simulink model "PMSM_Drive_custom_pwm_discrete"  (R2019b)
settings: Solver=VariableStepAuto  StartTime=0.0  StopTime=0.5  MaxStep=1e-6  RelTol=1e-3
undefined symbols (not defined in the file): Apd, f_sw, Tid, U_DC
libraries: coordinate_transformations x4, simulink x2, PE_components x1, controllers x1
settings Model: SimulationMode=accelerator  Creator=kissd  LastModifiedBy=kissd

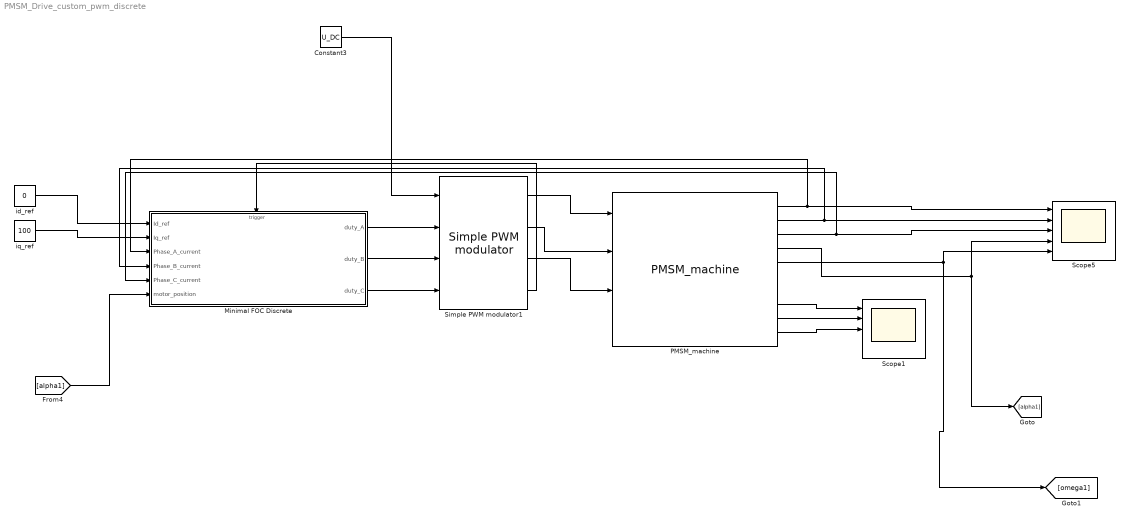
== system PMSM_Drive_custom_pwm_discrete ==
  Constant3 : Constant  Value=U_DC
  Minimal FOC Discrete : Subsystem  AncestorBlock=controllers/Minimal FOC Discrete
  PMSM_machine : PE_components/PMSM_machine  SystemSampleTime=-1  Latency=0  AutoFrameSizeCalculation=off
      link override Gain: Gain=1/Ld
      link override Gain1: Gain=Rs
      link override Gain2: Gain=Rs
      link override Gain4: Gain=1/Theta
      link override Gain7: Gain=3/2
      link override Integrator2: InitialCondition=0
      link override Sum2: Inputs=++-
  Scope1 : Scope  NumInputPorts=5
  Scope5 : Scope  NumInputPorts=5
  Simple PWM modulator1 : controllers/Simple PWM modulator  SystemSampleTime=-1  Latency=0  AutoFrameSizeCalculation=off
      link override Constant: Value=400
  id_ref : Constant  Value=0
  iq_ref : Constant  Value=100
  wires:
  PMSM_machine/2 -> Minimal FOC Discrete/4(Phase_B_current), Scope5/2
  PMSM_machine/3 -> Minimal FOC Discrete/5(Phase_C_current), Scope5/3
  PMSM_machine/1 -> Minimal FOC Discrete/3(Phase_A_current), Scope5/1
  PMSM_machine/4 -> [alpha1], Scope5/4
  PMSM_machine/5 -> [omega1], Scope5/5
  Constant3/1 -> Simple PWM modulator1/1
  Simple PWM modulator1/1 -> PMSM_machine/1
  Simple PWM modulator1/2 -> PMSM_machine/2
  Simple PWM modulator1/3 -> PMSM_machine/3
  PMSM_machine/8 -> Scope1/1
  PMSM_machine/9 -> Scope1/2
  PMSM_machine/10 -> Scope1/3
  id_ref/1 -> Minimal FOC Discrete/1(Id_ref)
  iq_ref/1 -> Minimal FOC Discrete/2(Iq_ref)
  [alpha1] -> Minimal FOC Discrete/6(motor_position)
  Minimal FOC Discrete/1(duty_A) -> Simple PWM modulator1/2
  Minimal FOC Discrete/2(duty_B) -> Simple PWM modulator1/3
  Minimal FOC Discrete/3(duty_C) -> Simple PWM modulator1/4
  Simple PWM modulator1/4 -> Minimal FOC Discrete/Trigger

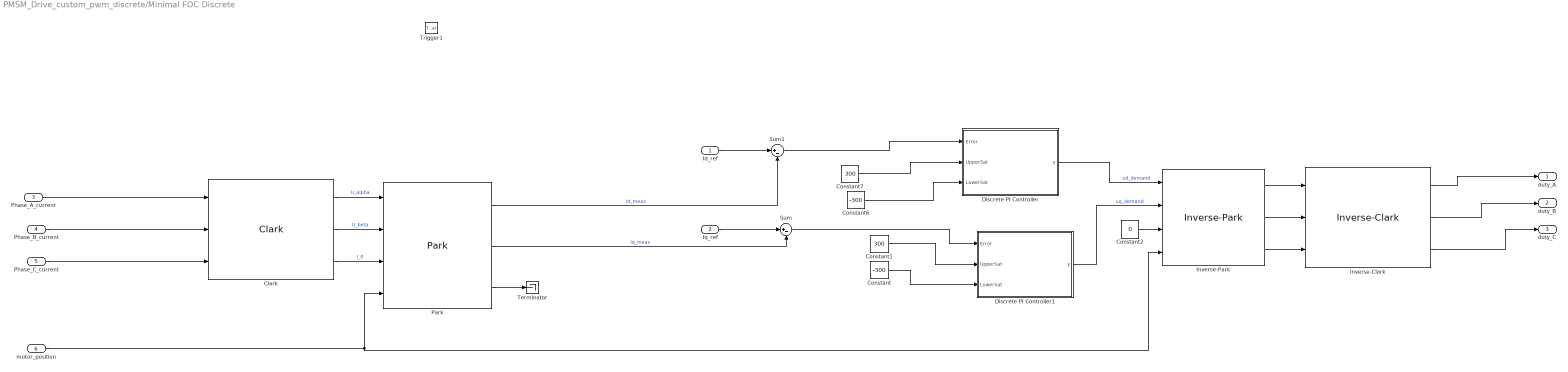
== system PMSM_Drive_custom_pwm_discrete/Minimal FOC Discrete ==
  Id_ref : Inport
  Iq_ref : Inport  Port=2
  Phase_A_current : Inport  Port=3
  Phase_B_current : Inport  Port=4
  Phase_C_current : Inport  Port=5
  motor_position : Inport  Port=6
  Trigger1 : TriggerPort  TriggerType=either  VariantControl=Variant  PortDimensions=1
  Clark : coordinate_transformations/Clark  SystemSampleTime=-1  Latency=0  AutoFrameSizeCalculation=off
  Constant : Constant  Value=-300
  Constant1 : Constant  Value=300
  Constant2 : Constant  Value=0
  Constant6 : Constant  Value=-300
  Constant7 : Constant  Value=300
  Discrete PI Controller : Subsystem  AncestorBlock=controllers/Discrete PI Controller  mask(Continous PI Controller){Apd=Apd, Tid=Tid, fs=f_sw}
      mask prompts: Apd "Proprotional Gain"; Tid "Integration Time"; fs "fsw"
      mask help: Continous PI Controller description.
  Discrete PI Controller1 : Subsystem  AncestorBlock=controllers/Discrete PI Controller  mask(Continous PI Controller){Apd=Apd, Tid=Tid, fs=f_sw}
      mask prompts: Apd "Proprotional Gain"; Tid "Integration Time"; fs "fsw"
      mask help: Continous PI Controller description.
  Inverse-Clark : coordinate_transformations/Inverse-Clark  SystemSampleTime=-1  Latency=0  AutoFrameSizeCalculation=off
  Inverse-Park : coordinate_transformations/Inverse-Park  SystemSampleTime=-1  Latency=0  AutoFrameSizeCalculation=off
  Park : coordinate_transformations/Park  SystemSampleTime=-1  Latency=0  AutoFrameSizeCalculation=off
  Sum : Sum  Inputs=|+-
  Sum1 : Sum  Inputs=|+-
  Terminator : Terminator
  duty_A : Outport
  duty_B : Outport  Port=2
  duty_C : Outport  Port=3
  wires:
  Discrete PI Controller1/1(y) -> Inverse-Park/2  "uq_demand"
  Inverse-Park/2 -> Inverse-Clark/2
  Inverse-Park/3 -> Inverse-Clark/3
  Park/2 -> Sum/2  "Iq_meas"
  Phase_C_current/1 -> Clark/3
  Constant7/1 -> Discrete PI Controller/2(UpperSat)
  Clark/1 -> Park/1  "U_alpha"
  Inverse-Clark/3 -> duty_C/1
  Constant1/1 -> Discrete PI Controller1/2(UpperSat)
  Sum/1 -> Discrete PI Controller1/1(Error)
  Inverse-Park/1 -> Inverse-Clark/1
  Constant6/1 -> Discrete PI Controller/3(LowerSat)
  motor_position/1 -> Park/4, Inverse-Park/4
  Park/1 -> Sum1/2  "Id_meas"
  Discrete PI Controller/1(y) -> Inverse-Park/1  "ud_demand"
  Constant/1 -> Discrete PI Controller1/3(LowerSat)
  Sum1/1 -> Discrete PI Controller/1(Error)
  Clark/2 -> Park/2  "U_beta"
  Iq_ref/1 -> Sum/1
  Clark/3 -> Park/3  "I_0"
  Park/3 -> Terminator/1
  Inverse-Clark/2 -> duty_B/1
  Id_ref/1 -> Sum1/1
  Inverse-Clark/1 -> duty_A/1
  Phase_B_current/1 -> Clark/2
  Phase_A_current/1 -> Clark/1
  Constant2/1 -> Inverse-Park/3

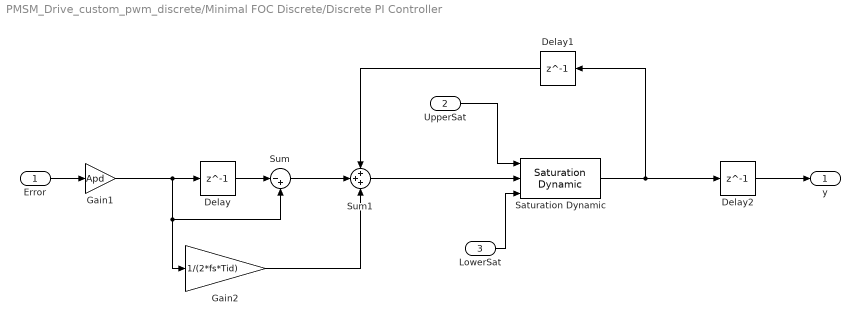
== system PMSM_Drive_custom_pwm_discrete/Minimal FOC Discrete/Discrete PI Controller ==
  Error : Inport
  UpperSat : Inport  Port=2
  LowerSat : Inport  Port=3
  Delay : Delay  DelayLength=1
  Delay1 : Delay  DelayLength=1
  Delay2 : Delay  DelayLength=1
  Gain1 : Gain  Gain=Apd
  Gain2 : Gain  Gain=1/(2*fs*Tid)
  Saturation Dynamic : simulink/Discontinuities/Saturation Dynamic  OutMin=[]  OutMax=[]  OutDataTypeStr=Inherit: Same as second input  OutDataType=fixdt(1, 16)  OutScaling=2^-10  DoSatur=off
  Sum : Sum  Inputs=|-+
  Sum1 : Sum  Inputs=+++
  y : Outport
  wires:
  Delay2/1 -> y/1
  Delay1/1 -> Sum1/1
  Gain2/1 -> Sum1/3
  Sum/1 -> Sum1/2
  Delay/1 -> Sum/1
  LowerSat/1 -> Saturation Dynamic/3
  UpperSat/1 -> Saturation Dynamic/1
  Saturation Dynamic/1 -> Delay2/1, Delay1/1
  Sum1/1 -> Saturation Dynamic/2
  Gain1/1 -> Delay/1, Sum/2, Gain2/1
  Error/1 -> Gain1/1

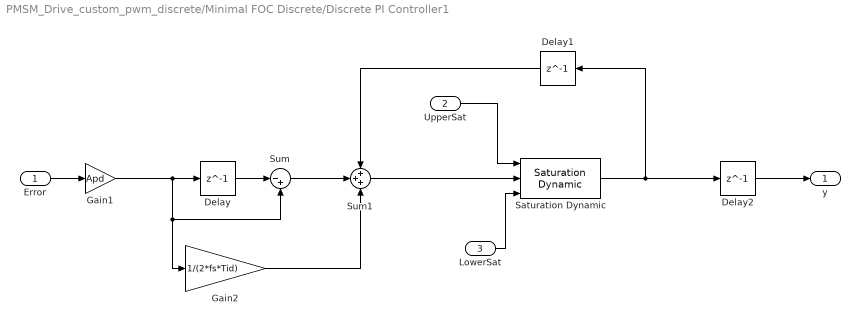
== system PMSM_Drive_custom_pwm_discrete/Minimal FOC Discrete/Discrete PI Controller1 ==
  Error : Inport
  UpperSat : Inport  Port=2
  LowerSat : Inport  Port=3
  Delay : Delay  DelayLength=1
  Delay1 : Delay  DelayLength=1
  Delay2 : Delay  DelayLength=1
  Gain1 : Gain  Gain=Apd
  Gain2 : Gain  Gain=1/(2*fs*Tid)
  Saturation Dynamic : simulink/Discontinuities/Saturation Dynamic  OutMin=[]  OutMax=[]  OutDataTypeStr=Inherit: Same as second input  OutDataType=fixdt(1, 16)  OutScaling=2^-10  DoSatur=off
  Sum : Sum  Inputs=|-+
  Sum1 : Sum  Inputs=+++
  y : Outport
  wires:
  Delay2/1 -> y/1
  Delay1/1 -> Sum1/1
  Gain2/1 -> Sum1/3
  Sum/1 -> Sum1/2
  Delay/1 -> Sum/1
  LowerSat/1 -> Saturation Dynamic/3
  UpperSat/1 -> Saturation Dynamic/1
  Saturation Dynamic/1 -> Delay2/1, Delay1/1
  Sum1/1 -> Saturation Dynamic/2
  Gain1/1 -> Delay/1, Sum/2, Gain2/1
  Error/1 -> Gain1/1
